simulink model "OpenLoopNashFormation"  (R2022b)
settings: Solver=VariableStepAuto  StartTime=0.0  StopTime=params.T  RelTol=1e-3
undefined symbols (not defined in the file or in its folder): dfc_opnash, graph, initial, model, params
settings Model: Creator=NTU  LastModifiedBy=NTU
settings DataIOCC: SaveState=on

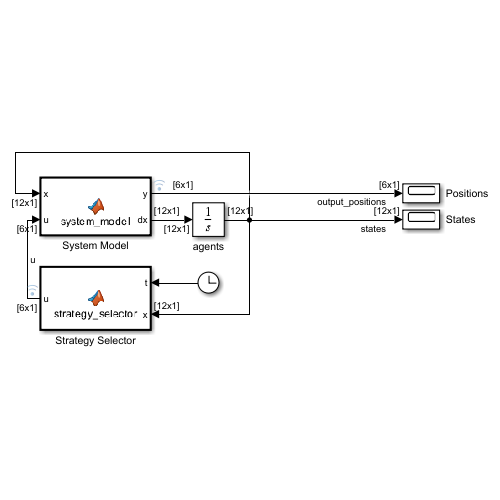
[thumbnail: Simulink's stored preview of the top-level diagram]
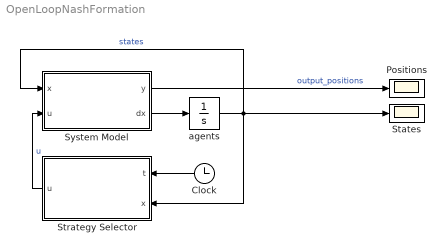
== system OpenLoopNashFormation ==
  Clock : Clock
  Positions : Scope
  States : Scope
  Strategy Selector : MATLAB Function  TreatAsAtomicUnit=on
  System Model : MATLAB Function  TreatAsAtomicUnit=on
  agents : Integrator  InitialCondition=initial.state  ContinuousStateAttributes='x'
  wires:
  System Model/2(dx) -> agents/1
  agents/1 -> Strategy Selector/2(x), System Model/1(x), States/1  "states"
  Strategy Selector/1(u) -> System Model/2(u)  "u"
  Clock/1 -> Strategy Selector/1(t)
  System Model/1(y) -> Positions/1  "output_positions"

== matlab function OpenLoopNashFormation/Strategy Selector ==
  data: t input; x input; u output; params parameter; initial parameter; model parameter; graph parameter; dfc_opnash parameter
function u = strategy_selector(t, x, params, initial, model, graph, dfc_opnash)
    u = open_loop_nash(t, x, params, initial, model, graph, dfc_opnash);
end

== matlab function OpenLoopNashFormation/System Model ==
  data: y output; x input; u input; dx output; params parameter; model parameter
function [y, dx] = system_model(x, u, params, model)
    n = params.n;
    m = params.m;
    p = params.p;
   
    dx = zeros(params.N * params.n, 1);
    y = zeros(params.N * params.m, 1);
    for i = 1:params.N
        [dx((i-1)*n+1 : i*n), y((i-1)*m+1 : i*m)] = ...
            agent_model(x((i-1)*n+1 : i*n), u((i-1)*p+1 : i*p), model);
    end
end
